simulink model "three_tank_nonlinear"  (R2020b)
settings: Solver=ode15s  StartTime=0.0  StopTime=2000  RelTol=1e-8  EnableMultiTasking=on
libraries: simulink x8, pid_lib x3
settings Model: Creator=Karl  LastModifiedBy=Fuzz4
settings DataIOCC: SaveFormat=Array  ReturnWorkspaceOutputs=off  OutputOption=SpecifiedOutputTimes  OutputTimes=[0:2000]
settings OptimizationCC: LifeSpan=inf
settings DebuggingCC: UnderspecifiedInitializationDetection=Classic  MergeDetectMultiDrivingBlocksExec=none  SFUnexpectedBacktrackingDiag=warning  SFNoUnconditionalDefaultTransitionDiag=warning  SFExecutionAtInitializationDiag=none  ArithmeticOperatorsInVariantConditions=warning
settings HardwareCC: ProdBitPerPointer=32  ProdBitPerSizeT=32  ProdBitPerPtrDiffT=32  ProdLargestAtomicFloat=None  ProdIntDivRoundTo=Undefined  ProdEndianess=Unspecified  ProdWordSize=32  ProdHWDeviceType=32-bit Generic
settings ModelReferenceCC: PropagateSignalLabelsOutOfModel=off
settings SFSimCC: SimUseLocalCustomCode=off  CustomCodeUndefinedFunction=UseInterfaceOnly
settings RTWCC: RTWUseLocalCustomCode=off
settings CodeAppCC: StateflowObjectComments=on
settings GRTTargetCC: TargetLangStandard=C89/C90 (ANSI)
settings ConfigComp: CovMetricSettings=dw  CovSaveCumulativeToWorkspaceVar=on  CovSaveSingleToWorkspaceVar=on  CovExternalEMLEnable=off

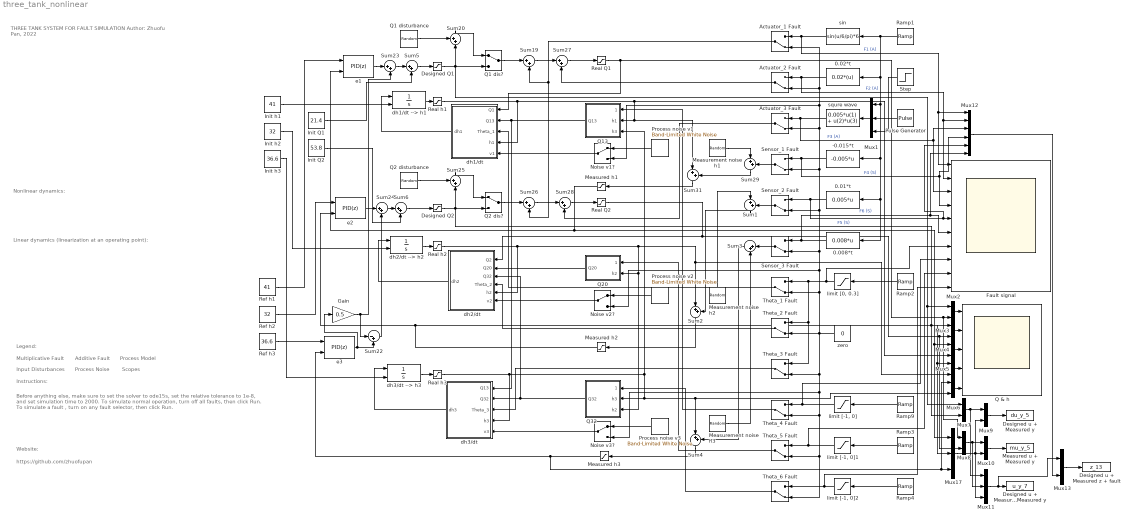
== system three_tank_nonlinear ==
  note: THREE TANK SYSTEM
      | FOR FAULT SIMULATION
      |
      | Author: Zhuofu Pan, 2022
  note: Multiplicative Fault
  note: Process Noise
  note: Process Model
  note: Input Disturbances
  note: Scopes
  note: Nonlinear dynamics:
  note: Linear dynamics
      | (linearization at an operating point):
  note: Before anything else, make sure to set the solver to ode15s, set the relative tolerance to 1e-8, and set simulation time to 2000.
      |
      | To simulate normal operation, turn off all faults, then click Run.
      |
      | To simulate a fault , turn on any fault selector, then click Run.
  note: Legend:
  note: Instructions:
  note: Website:
  note: https://github.com/zhuofupan
  note: Additive Fault
  " zero" : Constant  Value=0
  -0.015*t : Fcn  Expr=-0.005*u
  0.008*t : Fcn  Expr=0.008*u
  0.01*t : Fcn  Expr=0.005*u
  0.02*t : Fcn  Expr=0.02*(u)
  Actuator_1 Fault : ManualSwitch  CurrentSetting=0
  Actuator_2 Fault : ManualSwitch  CurrentSetting=0
  Actuator_3 Fault : ManualSwitch  CurrentSetting=0
  Designed Q1 : Saturate  UpperLimit=150  LowerLimit=0
  Designed Q2 : Saturate  UpperLimit=150  LowerLimit=0
  Designed u + Measured y : ToWorkspace  VariableName=du_y_5  SampleTime=-1
  Designed u + Measured u + Measured y : ToWorkspace  VariableName=u_y_7  SampleTime=-1
  Designed u + Measured z + fault : ToWorkspace  VariableName=z_13  SampleTime=-1
  Fault signal : Scope  NumInputPorts=10
  Gain : Gain  Gain=0.5
  Init Q1 : Constant  Value=21.4
  Init Q2 : Constant  Value=53.8
  Init h1 : Constant  Value=41
  Init h2 : Constant  Value=32
  Init h3 : Constant  Value=36.6
  Measured h1 : Saturate  UpperLimit=62  LowerLimit=0
  Measured h2 : Saturate  UpperLimit=62  LowerLimit=0
  Measured h3 : Saturate  UpperLimit=62  LowerLimit=0
  Measured u + Measured y : ToWorkspace  VariableName=mu_y_5  SampleTime=-1
  Measurement noise h1 : RandomNumber  Variance=0.02  Seed=randi(100000)
  Measurement noise h2 : RandomNumber  Variance=0.02  Seed=randi(100000)
  Measurement noise h3 : RandomNumber  Variance=0.02  Seed=randi(100000)
  Mux1 : Mux  Inputs=3
  Mux{2..10,13} (10 alike) : Mux  Inputs=2
  Mux11 : Mux  Inputs=3
  Mux12 : Mux  Inputs=6
  Mux17 : Mux  Inputs=3
  Noise v1? : ManualSwitch
  Noise v2? : ManualSwitch
  Noise v3? : ManualSwitch
  Process noise v1 : simulink/Sources/Band-Limited White Noise  Cov=[1e-4]  Ts=1  seed=randi(100000)
  Process noise v2 : simulink/Sources/Band-Limited White Noise  Cov=[1e-4]  Ts=1  seed=randi(100000)
  Process noise v3 : simulink/Sources/Band-Limited White Noise  Cov=[1e-4]  Ts=1  seed=randi(100000)
  Pulse Generator : DiscretePulseGenerator  PulseType=Time based  Amplitude=5  Period=60  PulseWidth=80
  Q & h : Scope  NumInputPorts=5
  Q1 dis? : ManualSwitch
  Q1 disturbance : RandomNumber  Variance=0.05  Seed=randi(100000)  SampleTime=15
  Q13 : MATLAB Function  TreatAsAtomicUnit=on
  Q2 dis? : ManualSwitch
  Q2 disturbance : RandomNumber  Variance=0.02  Seed=randi(100000)  SampleTime=15
  Q20 : MATLAB Function  TreatAsAtomicUnit=on
  Q32 : MATLAB Function  TreatAsAtomicUnit=on
  Ramp1 : simulink/Sources/Ramp  slope=1  start=200  InitialOutput=0
  Ramp2 : simulink/Sources/Ramp  slope=0.00005  start=200  InitialOutput=0
  Ramp3 : simulink/Sources/Ramp  slope=-0.0003  start=200  InitialOutput=0
  Ramp4 : simulink/Sources/Ramp  slope=-0.0005  start=200  InitialOutput=0
  Ramp9 : simulink/Sources/Ramp  slope=-0.0002  start=200  InitialOutput=0
  Real Q1 : Saturate  UpperLimit=150  LowerLimit=0
  Real Q2 : Saturate  UpperLimit=150  LowerLimit=0
  Real h1 : Saturate  UpperLimit=62  LowerLimit=0
  Real h2 : Saturate  UpperLimit=62  LowerLimit=0
  Real h3 : Saturate  UpperLimit=62  LowerLimit=0
  Ref h1 : Constant  Value=41
  Ref h2 : Constant  Value=32
  Ref h3 : Constant  Value=36.6
  Sensor_1 Fault : ManualSwitch  CurrentSetting=0
  Sensor_2 Fault : ManualSwitch  CurrentSetting=0
  Sensor_3 Fault : ManualSwitch  CurrentSetting=0
  Step : Step  Time=200  SampleTime=1
  Sum{1..6,19,23..24,26..29,31} (14 alike) : Sum  Inputs=|++
  Sum20 : Sum  Inputs=++|
  Sum22 : Sum  Inputs=|-+
  Sum25 : Sum  Inputs=++|
  Theta_1 Fault : ManualSwitch  CurrentSetting=0
  Theta_2 Fault : ManualSwitch  CurrentSetting=0
  Theta_3 Fault : ManualSwitch  CurrentSetting=0
  Theta_4 Fault : ManualSwitch  CurrentSetting=0
  Theta_5 Fault : ManualSwitch  CurrentSetting=0
  Theta_6 Fault : ManualSwitch  CurrentSetting=0
  dh1/dt : MATLAB Function  TreatAsAtomicUnit=on
  dh1/dt --> h1 : Integrator  InitialConditionSource=external  InitialCondition=416.723084574301  LimitOutput=on  UpperSaturationLimit=62  LowerSaturationLimit=0
  dh2/dt : MATLAB Function  TreatAsAtomicUnit=on
  dh2/dt --> h2 : Integrator  InitialConditionSource=external  InitialCondition=416.723084574301  LimitOutput=on  UpperSaturationLimit=62  LowerSaturationLimit=0
  dh3/dt : MATLAB Function  TreatAsAtomicUnit=on
  dh3/dt --> h3 : Integrator  InitialConditionSource=external  InitialCondition=416.723084574301  LimitOutput=on  UpperSaturationLimit=62  LowerSaturationLimit=0
  e1 : pid_lib/PID Controller (2DOF)  Controller=PID  Form=Parallel  TimeDomain=Discrete-time  UseExternalTs=off  SampleTime=-1  IntegratorMethod=Forward Euler  FilterMethod=Forward Euler  ControllerParametersSource=internal  P=0.3  I=0.3  D=0  UseFilter=on  N=100  b=1  c=1  TunerSelectOption=Transfer Function Based (PID Tuner App)  InitialConditionSource=internal  InitialConditionForIntegrator=0  InitialConditionForFilter=0  DifferentiatorICPrevScaledInput=0  ExternalReset=none  TrackingMode=off  Kt=1  LimitOutput=off  SatLimitsSource=internal  UpperSaturationLimit=inf  LowerSaturationLimit=-inf  LinearizeAsGain=on  AntiWindupMode=none  Kb=1  POutMin=[]  POutMax=[]  IOutMin=[]  IOutMax=[]  DOutMin=[]  DOutMax=[]  NOutMin=[]  NOutMax=[]  bOutMin=[]  bOutMax=[]  cOutMin=[]  cOutMax=[]  SumOutMin=[]  SumOutMax=[]  SaturationOutMin=[]  SaturationOutMax=[]  PParamMin=[]  PParamMax=[]  IParamMin=[]  IParamMax=[]  DParamMin=[]  DParamMax=[]  NParamMin=[]  NParamMax=[]  bParamMin=[]  bParamMax=[]  cParamMin=[]  cParamMax=[]  KbParamMin=[]  KbParamMax=[]  KtParamMin=[]  KtParamMax=[]  KbOutMin=[]  KbOutMax=[]  KtOutMin=[]  KtOutMax=[]  IntegratorOutMin=[]  IntegratorOutMax=[]  FilterOutMin=[]  FilterOutMax=[]  SumI1OutMin=[]  SumI1OutMax=[]  SumI2OutMin=[]  SumI2OutMax=[]  SumI3OutMin=[]  SumI3OutMax=[]  SumI4OutMin=[]  SumI4OutMax=[]  SumDOutMin=[]  SumDOutMax=[]  Sum1OutMin=[]  Sum1OutMax=[]  Sum2OutMin=[]  Sum2OutMax=[]  Sum3OutMin=[]  Sum3OutMax=[]  DifferentiatorOutMin=[]  DifferentiatorOutMax=[]  FilterDiffOutCoefMin=[]  FilterDiffOutCoefMax=[]  ReciprocalOutMin=[]  ReciprocalOutMax=[]  SumDenOutMin=[]  SumDenOutMax=[]  SumNumOutMin=[]  SumNumOutMax=[]  DivideOutMin=[]  DivideOutMax=[]  UdiffTsProdOutMin=[]  UdiffTsProdOutMax=[]  NTsProdOutMin=[]  NTsProdOutMax=[]  UintegralTsProdOutMin=[]  UintegralTsProdOutMax=[]  UngainTsProdOutMin=[]  UngainTsProdOutMax=[]  IntegratorContinuousStateAttributes=''  IntegratorStateMustResolveToSignalObject=off  IntegratorRTWStateStorageClass=Auto  FilterContinuousStateAttributes=''  FilterStateMustResolveToSignalObject=off  FilterRTWStateStorageClass=Auto  ParallelPVariant=InternalParameters  IdealPVariant=Disabled  IVariant=InternalParameters  DVariant=InternalParameters  bVariant=InternalParameters  cVariant=InternalParameters  IntegratorVariant=Discrete  SatVariant=Disabled  AWVariant=Passthrough  PCopyVariant=Disabled  TRVariant=Disabled  FdbkBlocksVariant=Forward  IdealPFdbkVariant=Disabled  SatFdbkVariant=Disabled  DerivativeFilterVariant=ForwardEulerFilter  NVariant=InternalParameters  NCopyVariant=Disabled  FilterICVariant=InternalICsFilter  IntegratorICVariant=InternalICs  ExternalResetVariant=Disabled  TRSumVariant=Passthrough  SumFdbkVariant=Disabled  SumVariant=Sum_PID  TsampFilterVariant=InternalTs  TsampNgainVariant=Passthrough  TsampIntegralVariant=Passthrough  ExternalSaturationOutDataTypeStr=Inherit: Same as second input
      settings: SourceProductBaseCode=SL
  e2 : pid_lib/PID Controller (2DOF)  Controller=PID  Form=Parallel  TimeDomain=Discrete-time  UseExternalTs=off  SampleTime=-1  IntegratorMethod=Forward Euler  FilterMethod=Forward Euler  ControllerParametersSource=internal  P=0.2  I=0.2  D=0  UseFilter=on  N=100  b=1  c=1  TunerSelectOption=Transfer Function Based (PID Tuner App)  InitialConditionSource=internal  InitialConditionForIntegrator=0  InitialConditionForFilter=0  DifferentiatorICPrevScaledInput=0  ExternalReset=none  TrackingMode=off  Kt=1  LimitOutput=off  SatLimitsSource=internal  UpperSaturationLimit=inf  LowerSaturationLimit=-inf  LinearizeAsGain=on  AntiWindupMode=none  Kb=1  POutMin=[]  POutMax=[]  IOutMin=[]  IOutMax=[]  DOutMin=[]  DOutMax=[]  NOutMin=[]  NOutMax=[]  bOutMin=[]  bOutMax=[]  cOutMin=[]  cOutMax=[]  SumOutMin=[]  SumOutMax=[]  SaturationOutMin=[]  SaturationOutMax=[]  PParamMin=[]  PParamMax=[]  IParamMin=[]  IParamMax=[]  DParamMin=[]  DParamMax=[]  NParamMin=[]  NParamMax=[]  bParamMin=[]  bParamMax=[]  cParamMin=[]  cParamMax=[]  KbParamMin=[]  KbParamMax=[]  KtParamMin=[]  KtParamMax=[]  KbOutMin=[]  KbOutMax=[]  KtOutMin=[]  KtOutMax=[]  IntegratorOutMin=[]  IntegratorOutMax=[]  FilterOutMin=[]  FilterOutMax=[]  SumI1OutMin=[]  SumI1OutMax=[]  SumI2OutMin=[]  SumI2OutMax=[]  SumI3OutMin=[]  SumI3OutMax=[]  SumI4OutMin=[]  SumI4OutMax=[]  SumDOutMin=[]  SumDOutMax=[]  Sum1OutMin=[]  Sum1OutMax=[]  Sum2OutMin=[]  Sum2OutMax=[]  Sum3OutMin=[]  Sum3OutMax=[]  DifferentiatorOutMin=[]  DifferentiatorOutMax=[]  FilterDiffOutCoefMin=[]  FilterDiffOutCoefMax=[]  ReciprocalOutMin=[]  ReciprocalOutMax=[]  SumDenOutMin=[]  SumDenOutMax=[]  SumNumOutMin=[]  SumNumOutMax=[]  DivideOutMin=[]  DivideOutMax=[]  UdiffTsProdOutMin=[]  UdiffTsProdOutMax=[]  NTsProdOutMin=[]  NTsProdOutMax=[]  UintegralTsProdOutMin=[]  UintegralTsProdOutMax=[]  UngainTsProdOutMin=[]  UngainTsProdOutMax=[]  IntegratorContinuousStateAttributes=''  IntegratorStateMustResolveToSignalObject=off  IntegratorRTWStateStorageClass=Auto  FilterContinuousStateAttributes=''  FilterStateMustResolveToSignalObject=off  FilterRTWStateStorageClass=Auto  ParallelPVariant=InternalParameters  IdealPVariant=Disabled  IVariant=InternalParameters  DVariant=InternalParameters  bVariant=InternalParameters  cVariant=InternalParameters  IntegratorVariant=Discrete  SatVariant=Disabled  AWVariant=Passthrough  PCopyVariant=Disabled  TRVariant=Disabled  FdbkBlocksVariant=Forward  IdealPFdbkVariant=Disabled  SatFdbkVariant=Disabled  DerivativeFilterVariant=ForwardEulerFilter  NVariant=InternalParameters  NCopyVariant=Disabled  FilterICVariant=InternalICsFilter  IntegratorICVariant=InternalICs  ExternalResetVariant=Disabled  TRSumVariant=Passthrough  SumFdbkVariant=Disabled  SumVariant=Sum_PID  TsampFilterVariant=InternalTs  TsampNgainVariant=Passthrough  TsampIntegralVariant=Passthrough  ExternalSaturationOutDataTypeStr=Inherit: Same as second input
      settings: SourceProductBaseCode=SL
  e3 : pid_lib/PID Controller (2DOF)  Controller=PID  Form=Parallel  TimeDomain=Discrete-time  UseExternalTs=off  SampleTime=-1  IntegratorMethod=Forward Euler  FilterMethod=Forward Euler  ControllerParametersSource=internal  P=0.1  I=0.1  D=0  UseFilter=on  N=100  b=1  c=1  TunerSelectOption=Transfer Function Based (PID Tuner App)  InitialConditionSource=internal  InitialConditionForIntegrator=0  InitialConditionForFilter=0  DifferentiatorICPrevScaledInput=0  ExternalReset=none  TrackingMode=off  Kt=1  LimitOutput=off  SatLimitsSource=internal  UpperSaturationLimit=inf  LowerSaturationLimit=-inf  LinearizeAsGain=on  AntiWindupMode=none  Kb=1  POutMin=[]  POutMax=[]  IOutMin=[]  IOutMax=[]  DOutMin=[]  DOutMax=[]  NOutMin=[]  NOutMax=[]  bOutMin=[]  bOutMax=[]  cOutMin=[]  cOutMax=[]  SumOutMin=[]  SumOutMax=[]  SaturationOutMin=[]  SaturationOutMax=[]  PParamMin=[]  PParamMax=[]  IParamMin=[]  IParamMax=[]  DParamMin=[]  DParamMax=[]  NParamMin=[]  NParamMax=[]  bParamMin=[]  bParamMax=[]  cParamMin=[]  cParamMax=[]  KbParamMin=[]  KbParamMax=[]  KtParamMin=[]  KtParamMax=[]  KbOutMin=[]  KbOutMax=[]  KtOutMin=[]  KtOutMax=[]  IntegratorOutMin=[]  IntegratorOutMax=[]  FilterOutMin=[]  FilterOutMax=[]  SumI1OutMin=[]  SumI1OutMax=[]  SumI2OutMin=[]  SumI2OutMax=[]  SumI3OutMin=[]  SumI3OutMax=[]  SumI4OutMin=[]  SumI4OutMax=[]  SumDOutMin=[]  SumDOutMax=[]  Sum1OutMin=[]  Sum1OutMax=[]  Sum2OutMin=[]  Sum2OutMax=[]  Sum3OutMin=[]  Sum3OutMax=[]  DifferentiatorOutMin=[]  DifferentiatorOutMax=[]  FilterDiffOutCoefMin=[]  FilterDiffOutCoefMax=[]  ReciprocalOutMin=[]  ReciprocalOutMax=[]  SumDenOutMin=[]  SumDenOutMax=[]  SumNumOutMin=[]  SumNumOutMax=[]  DivideOutMin=[]  DivideOutMax=[]  UdiffTsProdOutMin=[]  UdiffTsProdOutMax=[]  NTsProdOutMin=[]  NTsProdOutMax=[]  UintegralTsProdOutMin=[]  UintegralTsProdOutMax=[]  UngainTsProdOutMin=[]  UngainTsProdOutMax=[]  IntegratorContinuousStateAttributes=''  IntegratorStateMustResolveToSignalObject=off  IntegratorRTWStateStorageClass=Auto  FilterContinuousStateAttributes=''  FilterStateMustResolveToSignalObject=off  FilterRTWStateStorageClass=Auto  ParallelPVariant=InternalParameters  IdealPVariant=Disabled  IVariant=InternalParameters  DVariant=InternalParameters  bVariant=InternalParameters  cVariant=InternalParameters  IntegratorVariant=Discrete  SatVariant=Disabled  AWVariant=Passthrough  PCopyVariant=Disabled  TRVariant=Disabled  FdbkBlocksVariant=Forward  IdealPFdbkVariant=Disabled  SatFdbkVariant=Disabled  DerivativeFilterVariant=ForwardEulerFilter  NVariant=InternalParameters  NCopyVariant=Disabled  FilterICVariant=InternalICsFilter  IntegratorICVariant=InternalICs  ExternalResetVariant=Disabled  TRSumVariant=Passthrough  SumFdbkVariant=Disabled  SumVariant=Sum_PID  TsampFilterVariant=InternalTs  TsampNgainVariant=Passthrough  TsampIntegralVariant=Passthrough  ExternalSaturationOutDataTypeStr=Inherit: Same as second input
      settings: SourceProductBaseCode=SL
  "limit [-1, 0]" : Saturate  UpperLimit=0  LowerLimit=-1
  "limit [-1, 0]1" : Saturate  UpperLimit=0  LowerLimit=-1
  "limit [-1, 0]2" : Saturate  UpperLimit=0  LowerLimit=-1
  "limit [0, 0.3]" : Saturate  UpperLimit=0.3  LowerLimit=0
  sin : Fcn  Expr=sin(u/6/pi)*6
  squre wave : Fcn  Expr=0.005*u(1) + u(2)*u(3)
  wires:
  Theta_4 Fault/1 -> Q13/1(Theta_4)
  Theta_6 Fault/1 -> Q32/1(Theta_6)
  Q1 dis?/1 -> Sum19/1
  Theta_1 Fault/1 -> dh1/dt/3(Theta_1)
  Real h1/1 -> dh1/dt/4(h1), Mux4/2, Sum31/1, Q13/2(h1)
  Theta_5 Fault/1 -> Q20/1(Theta_5)
  Noise v1?/1 -> dh1/dt/5(v1)
  Sum28/1 -> Real Q2/1
  Q32/1(Q32) -> dh2/dt/3(Q32), dh3/dt/2(Q32)
  Q20/1(Q20) -> dh2/dt/2(Q20)
  Theta_2 Fault/1 -> dh2/dt/4(Theta_2)
  Real h2/1 -> dh2/dt/5(h2), Mux5/2, Sum2/1, Q20/2(h2), Q32/3(h2)
  Noise v2?/1 -> dh2/dt/6(v2)
  Q13/1(Q13) -> dh3/dt/1(Q13), dh1/dt/2(Q13)
  Theta_3 Fault/1 -> dh3/dt/3(Theta_3)
  Noise v3?/1 -> dh3/dt/5(v3)
  dh3/dt/1(dh3) -> dh3/dt --> h3/1
  dh3/dt --> h3/1 -> Real h3/1
  dh2/dt/1(dh2) -> dh2/dt --> h2/1
  dh1/dt/1(dh1) -> dh1/dt --> h1/1
  Ramp2/1 -> "limit [0, 0.3]"/1
  Process noise v2/1 -> Noise v2?/1
  Process noise v3/1 -> Noise v3?/1
  Process noise v1/1 -> Noise v1?/1
  Sum20/1 -> Q1 dis?/1
  Q1 disturbance/1 -> Sum20/1
  Ref h3/1 -> e3/1
  Ramp9/1 -> "limit [-1, 0]"/1
  Ref h2/1 -> e2/1
  Ref h1/1 -> e1/1
  e1/1 -> Sum23/1
  e3/1 -> Sum22/2, Gain/1
  Gain/1 -> Sum23/2, Sum22/1
  Sum22/1 -> Sum24/2
  e2/1 -> Sum24/1
  Init h1/1 -> dh1/dt --> h1/2
  Init h2/1 -> dh2/dt --> h2/2
  Init h3/1 -> dh3/dt --> h3/2
  Designed Q1/1 -> Mux2/1, Mux7/1, Sum20/2, Q1 dis?/2
  Sum25/1 -> Q2 dis?/1
  Q2 disturbance/1 -> Sum25/1
  Designed Q2/1 -> Sum25/2, Mux3/1, Mux7/2, Q2 dis?/2
  Actuator_1 Fault/1 -> Sum19/2, Sum26/2
  Sum27/1 -> Real Q1/1
  Q2 dis?/1 -> Sum26/1
  Sum19/1 -> Sum27/1
  Actuator_2 Fault/1 -> Sum27/2
  Sum26/1 -> Sum28/1
  Actuator_3 Fault/1 -> Sum28/2
  Sensor_1 Fault/1 -> Sum29/2
  Sum29/1 -> Sum31/2
  Measurement noise h2/1 -> Sum1/1
  Measurement noise h1/1 -> Sum29/1
  Sum31/1 -> Measured h1/1
  Real Q1/1 -> dh1/dt/1(Q1), Mux8/1, Mux2/2
  Real Q2/1 -> dh2/dt/1(Q2), Mux3/2, Mux8/2
  Mux7/1 -> Mux9/1, Mux11/1
  Measured h1/1 -> e1/2, Mux17/1, Mux4/1
  Ramp1/1 -> 0.008*t/1, 0.01*t/1, -0.015*t/1, Mux1/1, 0.02*t/1, sin/1
  Sum23/1 -> Sum5/1
  Sum24/1 -> Sum6/1
  Sensor_2 Fault/1 -> Sum1/2
  Sum2/1 -> Measured h2/1
  Measured h2/1 -> Mux17/2, Mux5/1, e2/2
  Sum1/1 -> Sum2/2
  Sensor_3 Fault/1 -> Sum3/1
  Measurement noise h3/1 -> Sum3/2
  Sum4/1 -> Measured h3/1
  Measured h3/1 -> Mux6/1, Mux17/3, e3/2
  Sum3/1 -> Sum4/2
  "limit [0, 0.3]"/1 -> Theta_1 Fault/1, Theta_3 Fault/1, Theta_2 Fault/1, Fault signal/7
  "limit [-1, 0]"/1 -> Theta_4 Fault/1, Fault signal/8
  sin/1 -> Fault signal/1, Mux12/1, Actuator_1 Fault/1  "F1 (A)"
  0.02*t/1 -> Mux12/2, Fault signal/2, Actuator_2 Fault/1  "F2 (A)"
  squre wave/1 -> Mux12/3, Fault signal/3, Actuator_3 Fault/1  "F3 (A)"
  -0.015*t/1 -> Sensor_1 Fault/1, Mux12/4, Fault signal/4  "F4 (S)"
  0.01*t/1 -> Sensor_2 Fault/1, Mux12/5, Fault signal/5  "F5 (S)"
  0.008*t/1 -> Fault signal/6, Mux12/6, Sensor_3 Fault/1  "F6 (S)"
  " zero"/1 -> Theta_1 Fault/2, Actuator_1 Fault/2, Actuator_2 Fault/2, Noise v1?/2, Actuator_3 Fault/2, Sensor_1 Fault/2, Sensor_2 Fault/2, Sensor_3 Fault/2, Noise v2?/2, Theta_6 Fault/2, Theta_5 Fault/2, Theta_4 Fault/2, Noise v3?/2, Theta_3 Fault/2, Theta_2 Fault/2
  Mux1/1 -> squre wave/1
  Pulse Generator/1 -> Mux1/2
  Step/1 -> Mux1/3
  dh1/dt --> h1/1 -> Real h1/1
  dh2/dt --> h2/1 -> Real h2/1
  Real h3/1 -> dh3/dt/4(h3), Mux6/2, Sum4/1, Q32/2(h3), Q13/3(h3)
  Mux2/1 -> Q & h/1
  Mux3/1 -> Q & h/2
  Mux4/1 -> Q & h/3
  Mux5/1 -> Q & h/4
  Mux6/1 -> Q & h/5
  Sum5/1 -> Designed Q1/1
  Init Q1/1 -> Sum5/2
  Sum6/1 -> Designed Q2/1
  Init Q2/1 -> Sum6/2
  Ramp3/1 -> "limit [-1, 0]1"/1
  Ramp4/1 -> "limit [-1, 0]2"/1
  "limit [-1, 0]1"/1 -> Fault signal/9, Theta_5 Fault/1
  "limit [-1, 0]2"/1 -> Fault signal/10, Theta_6 Fault/1
  Mux17/1 -> Mux9/2, Mux10/2, Mux11/3
  Mux8/1 -> Mux10/1, Mux11/2
  Mux9/1 -> Designed u + Measured y/1
  Mux10/1 -> Measured u + Measured y/1
  Mux11/1 -> Mux13/1, Designed u + Measured u + Measured y/1
  Mux12/1 -> Mux13/2
  Mux13/1 -> Designed u + Measured z + fault/1

== matlab function three_tank_nonlinear/Q32 ==
  data: Theta_6 input; h3 input; h2 input; Q32 output
function Q32 = fcn(Theta_6, h3, h2)
Q32 = 0.45*0.5*(1+Theta_6) *sign(h3-h2)*sqrt(2*981*abs(h3-h2));
end

== matlab function three_tank_nonlinear/Q13 ==
  data: Theta_4 input; Q13 output; h1 input; h3 input
function Q13 = fcn(Theta_4, h1, h3)
Q13 = 0.46*0.5*(1+Theta_4) *sign(h1-h3)*sqrt(2*981*abs(h1-h3));
end

== matlab function three_tank_nonlinear/Q20 ==
  data: Theta_5 input; h2 input; Q20 output
function Q20 = fcn(Theta_5, h2)
Q20 = 0.6*0.5*(1+ Theta_5)*sqrt(2*981*h2);
end

== matlab function three_tank_nonlinear/dh1//dt ==
  data: Q1 input; dh1 output; Q13 input; Theta_1 input; h1 input; v1 input
function dh1 = fcn(Q1, Q13, Theta_1, h1, v1)
dh1 = (Q1 - Q13 - Theta_1*sqrt(2*981*h1 ))/154 + v1;
end

== matlab function three_tank_nonlinear/dh2//dt ==
  data: Q2 input; Q20 input; dh2 output; Q32 input; Theta_2 input; h2 input; v2 input
function dh2 = fcn(Q2, Q20, Q32, Theta_2, h2, v2)
dh2 = (Q2 + Q32 - Q20 - Theta_2*sqrt(2*981*h2) )/154 + v2;
end

== matlab function three_tank_nonlinear/dh3//dt ==
  data: Q13 input; dh3 output; Q32 input; Theta_3 input; h3 input; v3 input
function dh3 = fcn(Q13, Q32, Theta_3, h3, v3)
dh3 = (Q13 - Q32 - Theta_3*sqrt(2*981*h3) )/154 + v3;
end
